simulink model "P414_1_model02_comp"  (R2021a)
settings: Solver=VariableStepAuto  StartTime=0.0  StopTime=4  RelTol=1e-3
model workspace (MAT data in the model file):
  clima__A_c = 3295.16408265
  clima__A_f = 3100.53942116
  clima__G0 = [0.05; 0.00070738]
  clima__H = 7.9995824611
  clima__T0 = [287.15; 287.15; 287.15; 287.15]
  clima__T_ss = 280.150340169
  clima__alpha_c = 0.0100640347387
  clima__alpha_f = 0.0111385012129
  clima__alpha_i = 0.1
  clima__c_s = [1081 1081]
  clima__cd_c = 8736
  clima__d_c = 1.5
  clima__hour0 = 1
  clima__int_air_speed = 0.5
  clima__l_s = [0.1 0.1]
  clima__lam_s = [2.5 0.85]
  clima__minWindows = 0.299965865643
  clima__rhod_s = [2600 2500]
  clima__tau_c = 1
  crop__A_v = 2080
  crop__C = [0.01 0.001 0.01 0.01]
  crop__C_buf_max = 0.02
  crop__C_wv = 0.2
  crop__Chi_nutrients = [0.015625; 0.0104166666667; 0.00520833333333; 0.00208333333333; 0.00208333333333; 0.00104166666667; 0; 0]
  crop__N = [0; 0; 0; 0; 0; 0; 0; 0]
  crop__R = [0 0 0]
  crop__T_max_v = 40
  crop__T_max_v24 = 27
  crop__T_min_v = 6
  crop__T_min_v24 = 14
  crop__T_sum_end = 1035
  crop__T_v_start_fruit = 1100
  crop__Tsum = 0
  crop__Tv = 288
  crop__b_N_uptake = 0.5
  crop__c_fruit_g = 0.27
  crop__c_fruit_m = 2.3e-07
  crop__c_leaf_g = 0.28
  crop__c_leaf_m = 3.47e-07
  crop__c_stem_g = 0.3
  crop__c_stem_m = 1.47e-07
  crop__fraction_DM = 0.08
  crop__int_air_speed = 0.5
  crop__min_water_capacity = 0.1
  crop__plants_density = 2.1562
  crop__rg_fruit = 2e-07
  crop__rg_leaf = 9.5e-08
  crop__rg_stem = 7.4e-08
  crop__s_buforg_buf = -5000
  crop__s_max_T = 0.5793
  crop__s_max_T24 = 1.3904
  crop__s_min_T = -0.869
  crop__s_min_T24 = -1.1587
  heater__A_e = 0.0001
  heater__A_i = 0.008
  heater__T = 288
  heater__c = 5e-10
  heater__power = 60000000
  screen__Power = 100
  screen__Radthreshold = 900
  screen__beta = 2.23564167038e-14
  screen__gamma_max = 2.26308905438e-14
  screen__velocity = 0.333333333333
  subtrate__C_ws = 0.1
  subtrate__N = [0; 0; 0; 0; 0; 0; 0; 0]
  subtrate__Nmin_subs = 1e-09
  subtrate__Vmax_subs = 10
  subtrate__Vmin_subs = 0.01
  tomato__Cfruit0 = 0.001
  windows__AR = 19.9974923936
  windows__Power = 100
  windows__RadThreshold = 10
  windows__max_night = 10
  windows__tau = 600
values from neighbouring files (symbols this model uses):
  Tmax = 296    [P414_3_script.m]
  Tstart = 285.5    [P414_3_script.m]
libraries: HORTISIM x11
settings Model: DataDictionary=dic.sldd  ParameterArgumentNames=clima__A_c,clima__A_f  OrderedModelArguments=off  Creator=djoroya  LastModifiedBy=djoroya
settings SolverCC: MaxConsecutiveMinStep=2
settings DataIOCC: SaveFormat=StructureWithTime
settings HardwareCC: TargetBitPerLong=64  TargetBitPerPointer=64  TargetBitPerSizeT=64  TargetBitPerPtrDiffT=64  TargetLongLongMode=on  TargetIntDivRoundTo=Zero  TargetEndianess=LittleEndian  TargetWordSize=64  TargetHWDeviceType=MATLAB Host  ProdEqTarget=off
settings RTWCC: Description=Rapid Simulation Target  SystemTargetFile=rsim.tlc  TemplateMakefile=rsim_default_tmf
settings RSimTargetCC: TargetLangStandard=C99 (ISO)

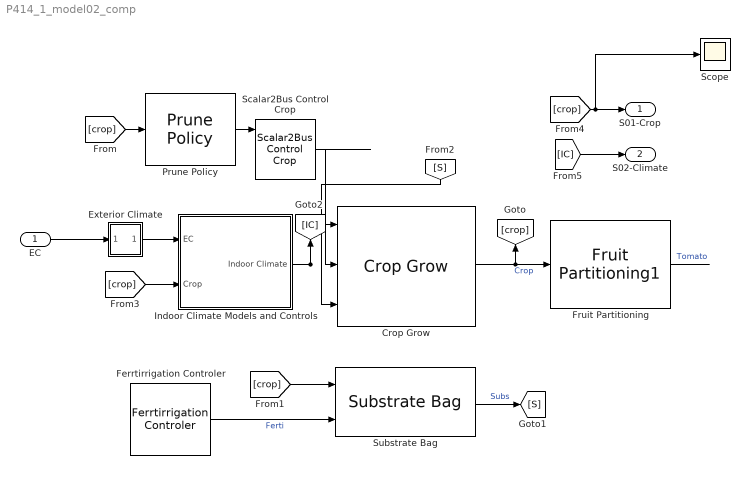
== system P414_1_model02_comp ==
  EC : Inport
  Crop Grow : HORTISIM/Horticulture/Models/Crop Grow  Chi_nutrients=crop__Chi_nutrients  A_v=crop__A_v  plants_density=crop__plants_density  fraction_DM=crop__fraction_DM  min_water_capacity=crop__min_water_capacity  C_buf_max=crop__C_buf_max  T_v_start_fruit=crop__T_v_start_fruit  int_air_speed=crop__int_air_speed  b_N_uptake=crop__b_N_uptake  Tv=crop__Tv  C=crop__C  R=crop__R  Tsum=crop__Tsum  C_wv=crop__C_wv  N=crop__N  rg_fruit=crop__rg_fruit  c_fruit_m=crop__c_fruit_m  c_fruit_g=crop__c_fruit_g  rg_leaf=crop__rg_leaf  c_leaf_m=crop__c_leaf_m  c_leaf_g=crop__c_leaf_g  rg_stem=crop__rg_stem  c_stem_m=crop__c_stem_m  c_stem_g=crop__c_stem_g  T_max_v=crop__T_max_v  s_max_T=crop__s_max_T  s_min_T=crop__s_min_T  s_buforg_buf=crop__s_buforg_buf  T_sum_end=crop__T_sum_end  T_max_v24=crop__T_max_v24  T_min_v24=crop__T_min_v24  s_min_T24=crop__s_min_T24  s_max_T24=crop__s_max_T24  T_min_v=crop__T_min_v
      settings: SourceProductName=Horti Simulator
  Exterior Climate : Subsystem
  Ferrtirrigation Controler : HORTISIM/Horticulture/Controls/Ferrtirrigation  Controler  SystemSampleTime=-1  VariantActivationTime=update diagram  Latency=0  AutoFrameSizeCalculation=off
      settings: SourceProductName=Horti Simulator
  Fruit Partitioning : HORTISIM/Horticulture/Models/Fruit Partitioning1  Cfruit0=tomato__Cfruit0
      settings: SourceProductName=Horti Simulator
  Indoor Climate Models and Controls : Subsystem
  Prune Policy : HORTISIM/Horticulture/Controls/Prune Policy  SystemSampleTime=-1  VariantActivationTime=update diagram  Latency=0  AutoFrameSizeCalculation=off
      settings: SourceProductName=Horti Simulator
  Scalar2Bus Control Crop : HORTISIM/Other  Functions/Scalar2Bus Control Crop  SystemSampleTime=-1  VariantActivationTime=update diagram  Latency=0  AutoFrameSizeCalculation=off
      settings: SourceProductName=Horti Simulator
  Scope : Scope
  Substrate Bag : HORTISIM/Horticulture/Models/Substrate Bag  Vmax_subs=subtrate__Vmax_subs  Vmin_subs=subtrate__Vmin_subs  Nmin_subs=subtrate__Nmin_subs  C_ws=subtrate__C_ws  N=subtrate__N
      settings: SourceProductName=Horti Simulator
  S01-Crop : Outport
  S02-Climate : Outport  Port=2
  wires:
  Exterior Climate/1(EC) -> Indoor Climate Models and Controls/1(EC)
  Indoor Climate Models and Controls/1(Indoor Climate) -> [IC], Crop Grow/1
  Crop Grow/1 -> [crop], Fruit Partitioning/1  "Crop"
  Ferrtirrigation Controler/1 -> Substrate Bag/2  "Ferti"
  Scalar2Bus Control Crop/1 -> Crop Grow/2
  Prune Policy/1 -> Scalar2Bus Control Crop/1
  [crop] -> Prune Policy/1
  [crop] -> Substrate Bag/1
  Substrate Bag/1 -> [S]  "Subs"
  [S] -> Crop Grow/3
  [crop] -> Indoor Climate Models and Controls/2(Crop)
  Fruit Partitioning/1 -> ?  "Tomato"
  EC/1 -> Exterior Climate/1(In1)
  [IC] -> S02-Climate/1
  [crop] -> Scope/1, S01-Crop/1

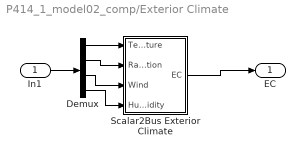
== system P414_1_model02_comp/Exterior Climate ==
  In1 : Inport
  Demux : Demux
  Scalar2Bus Exterior Climate : Subsystem
  EC : Outport
  wires:
  Demux/3 -> Scalar2Bus Exterior Climate/3(Wind)
  Demux/2 -> Scalar2Bus Exterior Climate/2(Radiation)
  Scalar2Bus Exterior Climate/1(EC) -> EC/1
  Demux/1 -> Scalar2Bus Exterior Climate/1(Temperature)
  Demux/4 -> Scalar2Bus Exterior Climate/4(Humidity)
  In1/1 -> Demux/1

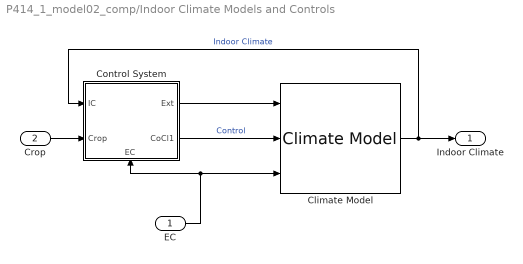
== system P414_1_model02_comp/Indoor Climate Models and Controls ==
  EC : Inport
  Crop : Inport  Port=2
  Climate Model : HORTISIM/Climate/Models/Climate Model  hour0=clima__hour0  G0=clima__G0  T0=clima__T0  H=clima__H  A_f=clima__A_f  A_c=clima__A_c  minWindows=clima__minWindows  lam_s=clima__lam_s  c_s=clima__c_s  l_s=clima__l_s  rhod_s=clima__rhod_s  int_air_speed=clima__int_air_speed  alpha_i=clima__alpha_i  alpha_c=clima__alpha_c  tau_c=clima__tau_c  alpha_f=clima__alpha_f  d_c=clima__d_c  cd_c=clima__cd_c  T_ss=clima__T_ss
      settings: SourceProductName=Horti Simulator
  Control System : Subsystem
      settings: PortSchema="{\"entries\":[{\"content\":{\"sides\":[{\"content\":{\"connectorIds\":[\"In1\",\"In2\"]},\"type\":\"ConnectorPlacement.EquallySpacedRectSide\",\"uuid\":\"7d0146e2-a53b-49ab-a7f4-04cd7ef00b9a\"},{\"content\":{\"connectorIds\":[\"Out1\",\"Out2\"],\"side\":\"RIGHT\"},\"type\":\"ConnectorPlacement.EquallySpacedRectSide\",\"uuid\":\"fee587e2-4b5c-4140-8904-07609d427593\"},{\"content\":{\"connectorIds\":[],\"side\":\"TOP\"},\"type\":\"ConnectorPlacement.EquallySpacedRectSide\",\"uuid\":\"52e767bc-1595-40ac-996f-44c9eedd0a08\"},{\"content\":{\"connectorIds\":[\"In3\"],\"side\":\"BOTTOM\"},\"type\":\"ConnectorPlacement.EquallySpacedRectSide\",\"uuid\":\"c629db5c-cfe6-4bd1-aeb9-7fba46dde396\"}]},\"type\":\"ConnectorPlacement.EquallySpacedConnector\",\"uuid\":\"268fde01-3c08-4d62-bfbb-fc94284c5cdd\"}],\"packageUris\":[\"http://schema.mathworks.com/mf0/Connector/R2020b\"],\"version\":\"1.0\"}"
  Indoor Climate : Outport
  wires:
  Climate Model/1 -> Indoor Climate/1, Control System/1(IC)  "Indoor Climate"
  Control System/2(CoCl1) -> Climate Model/2  "Control"
  Control System/1(Ext) -> Climate Model/1
  EC/1 -> Control System/3(EC), Climate Model/3
  Crop/1 -> Control System/2(Crop)

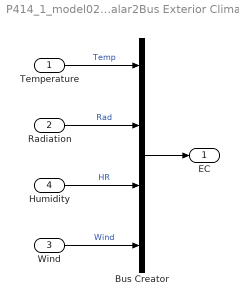
== system P414_1_model02_comp/Exterior Climate/Scalar2Bus Exterior Climate ==
  Temperature : Inport
  Radiation : Inport  Port=2
  Wind : Inport  Port=3
  Humidity : Inport  Port=4
  Bus Creator : BusCreator  Inputs=4
  EC : Outport
  wires:
  Humidity/1 -> Bus Creator/3  "HR"
  Wind/1 -> Bus Creator/4  "Wind"
  Temperature/1 -> Bus Creator/1  "Temp"
  Bus Creator/1 -> EC/1
  Radiation/1 -> Bus Creator/2  "Rad"

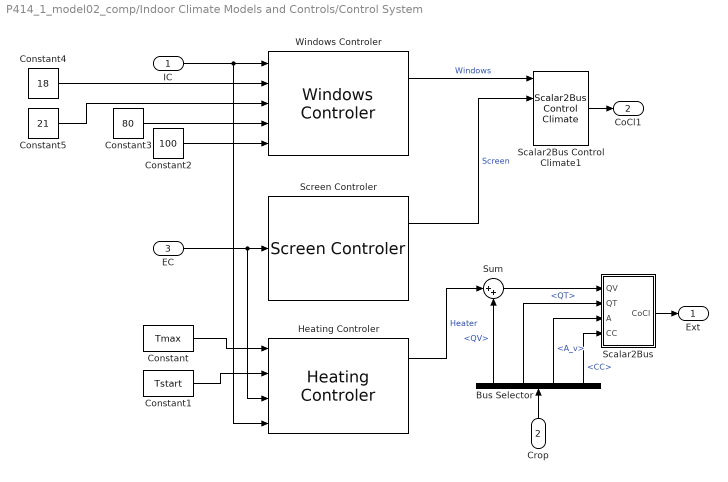
== system P414_1_model02_comp/Indoor Climate Models and Controls/Control System ==
  IC : Inport
  Crop : Inport  Port=2
  EC : Inport  Port=3
  Bus Selector : BusSelector  OutputSignals=HeatVars.QV,HeatVars.QT,A_v,CC
  Constant : Constant  Value=Tmax
  Constant1 : Constant  Value=Tstart
  Constant2 : Constant  Value=100
  Constant3 : Constant  Value=80
  Constant4 : Constant  Value=18
  Constant5 : Constant  Value=21
  Heating Controler : HORTISIM/Climate/Controls/Heating Controler  T=heater__T  power=heater__power  A_e=heater__A_e  A_i=heater__A_i  c=heater__c
      settings: SourceProductName=Horti Simulator
  "Scalar2Bus " : Subsystem
  Scalar2Bus Control Climate1 : HORTISIM/Other  Functions/Scalar2Bus  Control Climate  SystemSampleTime=-1  VariantActivationTime=update diagram  Latency=0  AutoFrameSizeCalculation=off
      settings: SourceProductName=Horti Simulator
  Screen Controler : HORTISIM/Climate/Controls/Screen Controler  Radthreshold=screen__Radthreshold  velocity=screen__velocity  Power=screen__Power  gamma_max=screen__gamma_max  beta=screen__beta
      settings: SourceProductName=Horti Simulator
  Sum : Sum  Inputs=|++
  Windows Controler : HORTISIM/Climate/Controls/Windows Controler  Power=windows__Power  max_night=windows__max_night  tau=windows__tau  RadThreshold=windows__RadThreshold  AR=windows__AR
      settings: SourceProductName=Horti Simulator
  Ext : Outport
  CoCl1 : Outport  Port=2
  wires:
  EC/1 -> Heating Controler/3, Screen Controler/1
  "Scalar2Bus "/1(CoCl) -> Ext/1
  Constant1/1 -> Heating Controler/2
  Constant/1 -> Heating Controler/1
  Windows Controler/1 -> Scalar2Bus Control Climate1/1  "Windows"
  Scalar2Bus Control Climate1/1 -> CoCl1/1
  Screen Controler/1 -> Scalar2Bus Control Climate1/2  "Screen"
  IC/1 -> Heating Controler/4, Windows Controler/1
  Constant2/1 -> Windows Controler/5
  Constant3/1 -> Windows Controler/4
  Constant4/1 -> Windows Controler/2
  Constant5/1 -> Windows Controler/3
  Crop/1 -> Bus Selector/1
  Sum/1 -> "Scalar2Bus "/1(QV)
  Bus Selector/1 -> Sum/2  "<QV>"
  Heating Controler/1 -> Sum/1  "Heater"
  Bus Selector/2 -> "Scalar2Bus "/2(QT)  "<QT>"
  Bus Selector/3 -> "Scalar2Bus "/3(A)  "<A_v>"
  Bus Selector/4 -> "Scalar2Bus "/4(CC)  "<CC>"

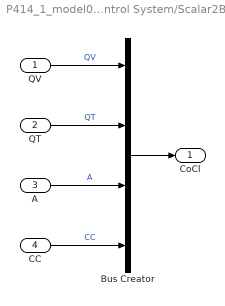
== system P414_1_model02_comp/Indoor Climate Models and Controls/Control System/Scalar2Bus  ==
  QV : Inport
  QT : Inport  Port=2
  A : Inport  Port=3
  CC : Inport  Port=4
  Bus Creator : BusCreator  Inputs=4
  CoCl : Outport
  wires:
  A/1 -> Bus Creator/3  "A"
  CC/1 -> Bus Creator/4  "CC"
  QV/1 -> Bus Creator/1  "QV"
  Bus Creator/1 -> CoCl/1
  QT/1 -> Bus Creator/2  "QT"
